simulink library "fm_lib"  (R2014a)
settings: Solver=ode45  SolverMode=SingleTasking  StartTime=0.0  StopTime=10.0  RelTol=1e-3
(part 2 of 2)

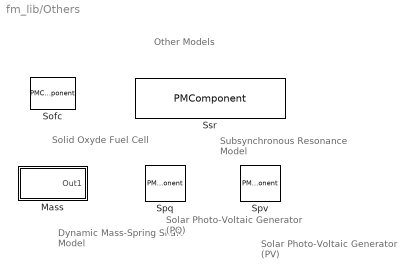
== system fm_lib/Others ==
  note: Other Models
  note: Subsynchronous
      | Resonance Model
  note: Solid Oxyde
      | Fuel Cell
  note: Dynamic Mass-Spring
      | Shaft Model
  note: Solar Photo-Voltaic
      | Generator (PQ)
  note: Solar Photo-Voltaic
      | Generator (PV)
  Mass : Subsystem  Tag=PSATblock  Description=Sparse Dynamic Component  mask(Mass){p2_3_4_5q=[0.6695  1.4612  1.6307  0.0903], p6_7_8_9q=[0.518  0.224  0.224  0.145], p10_11_12_13q=[0.0518  0.0224  0.0224  0.0145], p14_15_16_17q=[33.07  28.59  44.68  21.98], in=0, p18q=on}
      mask prompts: p2_3_4_5q "HP, IP, LP and EX inertiae [1/s 1/s 1/s 1/s]"; p6_7_8_9q "HP, IP, LP and EX damping [p.u. p.u. p.u. p.u.]"; p10_11_12_13q "D12, D23, D34 and D45 damping [p.u. p.u. p.u. p.u.]"; p14_15_16_17q "K12, K23, K34 and K45 coefficients"; in "Number of input signals"; p18q "Connected"
      mask help: This block defines a mechanical model for synchronous generator shaft.
      mask init:
      | fm_inout
      | [x,y] = fm_draw('circle');
      | [x1,y1] = fm_draw('semicircle');
      mask TypeOptions in: 0 | 1
      mask Callback p18q: fm_block
      mask Display: plot(-x1,y1,3+x,y,[0 3],[1 1],[0 3],[-1 -1],[3 5],[0 0])
  Sofc : PMComponent  Tag=PSATblock  Description=Sparse Dynamic Component  PhysicalDomain=psatdomain  LeftPortType=p1  RightPortType=p1  RConnTagsString=__newr0  mask(Sofc){p2_3q=[100  333.8], p4_13q=[0.8  5], p5_8_10q=[26.1  78.3  2.91], p6_9_11q=[8.43e-4  2.81e-4  2.52e-3], p7_17_12q=[0.996e-6  0.126  1.145], p14_15_16q=[0.85  0.9  0.8], p18_19q=[384  1.18], p20q=1273, p26q=0.1, p27_28q=[100  10], p29_30q=[1.2  0.8], p25q=0, p31q=on}
      mask prompts: p2_3q "DC Power and Voltage Rating [MW, kV]"; p4_13q "Electrical and fuel processor response times (Te, Tf) [s, s]"; p5_8_10q "Response times TH2, TH2O and TO2 [s, s, s]"; p6_9_11q "Valve molar constants KH2, KH2O and KO2"; p7_17_12q "Constant Kr, ohmic loss [Ohm] and hydrogen to oxygen ratio rH_O"; p14_15_16q "Fuel optimization constants Uopt, Umax and Umin"; p18_19q "Number of cells N0 and ideal standard potential E0 [V]"; p20q "Gas absolute temperature T [K]"; p26q "Transformer reactance Xt [p.u.]"; p27_28q "Gain and Time constant for Voltage Control Km, Tm [p.u.  s]"; p29_30q "Max and Min tap ratio [p.u./p.u. p.u./p.u.]"; p25q "Control Mode: [0] costant current; [1] costant power"; p31q "Connected"
      mask help: This block defines a Solid Oxyde Fuel Cell:
      mask TypeOptions p25q: 1 | 0
      mask Callback p31q: fm_block
      mask Display:
      | plot([0 1 1 0 0],[0 0 1 1 0])
      | plot([0.1 0.1 0.3 0.3],[1 1.1 1.1 1])
      | plot([0.9 0.9 0.7 0.7],[1 1.1 1.1 1])
      | color('yellow')
      | plot([0.85 0.75],[0.85 0.85],[0.15 0.25],[0.85 0.85],[0.8 0.8],[0.8 0.9])
      | color('blue')
      | plot([0.85 0.65 0.65 0.85 0.85],[0.3 0.3 0.7 0.7 0.3])
      | plot([0.15 0.15],[0.3 0.7],[0.35 0.35],[0.3 0.7],[0.15 0.35],[0.5 0.5])
      | plot([0.55 0.45 0.45 0.55 0.55 0.45],[0.15 0.15 0.25 0.25 0.35 0.35])
  Spq : PMComponent  Tag=PSATblock  Description=Sparse Dynamic Component  PhysicalDomain=psatdomain  LeftPortType=p1  RightPortType=p1  RConnTagsString=__newr0  mask(Spq){p2_3q=[60  80], p4_5q=[15  15], p6q=on}
      mask prompts: p2_3q "Active and Reactive Power Rating [MW, MVar]"; p4_5q "Inverter response times (Tp, Tq) [s, s]"; p6q "Connected"
      mask help: This block defines a Solar Photo-Voltaic generator with constant PQ model.
      mask init:
      | [x,y] = fm_draw('circle');
      | [xc,yc] = fm_draw('S');
      mask Callback p6q: fm_block
      mask Display:
      | plot(x,y,[-0.25 -0.25],[-0.25 0.25])
      | color('blue')
      | plot(xc,yc)
  Spv : PMComponent  Tag=PSATblock  Description=Sparse Dynamic Component  PhysicalDomain=psatdomain  LeftPortType=p1  RightPortType=p1  RConnTagsString=__newr0  mask(Spv){p2_3q=[40  1.045], p4_5q=[0.015  0.015], p6_7q=[0.0868  50.9005], p8q=on}
      mask prompts: p2_3q "Active Power and Voltage References [MW, p.u.]"; p4_5q "Inverter response times (Tp, Tq) [s, s]"; p6_7q "Voltage PI Controller Gains (kv, ki)"; p8q "Connected"
      mask help:
      | This block defines a Solar Photo-Voltaic generator.
      | P_ref = const
      | V_ref = const
      mask init:
      | [x,y] = fm_draw('circle');
      | [x1,y1] = fm_draw('sunedge');
      | [xp,yp] = fm_draw('G');
      mask Callback p8q: fm_block
      mask Display:
      | plot(1.1*x,1.1*y,[-0.25 -0.25],[-0.25 0.25])
      | plot(1.5*x1,y1)
      | plot(-1.5*x1,y1)
      | plot(y1,1.5*x1)
      | plot(y1,-1.5*x1)
      | color('blue')
      | plot(0.5*xp,0.5*yp)
  Ssr : PMComponent  Tag=PSATblock  Description=Sparse Dynamic Component  PhysicalDomain=psatdomain  LeftPortType=p1  RightPortType=p1  RConnTagsString=__newr0  mask(SSR){p2_3_4q=[100   230  60], p5_6q=[1.79  1.71], p8_7q=[1.66  0.015], p13_12q=[1.70  0.01], p9_10_11q=[0.0165  0.30  0.05], p14_15_16_17_18q=[0.6695  1.4612  1.6307  1.5228  0.0903], p19_20_21_22_23q=[0.518  0.224  0.224  0.000  0.145], p24_25_26_27q=[33.07  28.59  44.68  21.98], p28q=on}
      mask prompts: p2_3_4q "Power, Voltage and Frequency Ratings [MVA, kV, Hz]"; p5_6q "Machine reactances Xd, Xq [p.u. p.u.]"; p8_7q "Armature parameters Xad, Ra [p.u. p.u.]"; p13_12q "D-axis parameters Xf, Rf [p.u. p.u.]"; p9_10_11q "Line parameters R, Xl, Xc [p.u. p.u. p.u.]"; p14_15_16_17_18q "Inertiae M (HP, IP, LP, rotor, EX)"; p19_20_21_22_23q "Dampings D (HP, IP, LP, rotor, EX)"; p24_25_26_27q "Shaft coefficients K12, K23, K34, K45"; p28q "Connected"
      mask help: This block defines a fourth order synchronous machine with shaft dynamics and compensated line.
      mask init:
      | [x,y] = fm_draw('circle');
      | [xg,yg] = fm_draw('G');
      | [xs,ys] = fm_draw('sinus');
      mask Callback p28q: fm_block
      mask Display:
      | plot(0,-50,450,50,[0 30 30 38 53 68 83 98 113 120 120 150],[0 0 0 25 -25 25 -25 25 -25 0 0 0],[0 23 23 24 28 34 40 47 52 55 56 54 51 51 47 46 48 51 57 64 70 75 79 79 77 74 74 70 69 71 75 80 87 93 99 102 103 101 97 97 94 93 94 98 104 110 117 122 125 126 126 150]+150,[0 0 1 11 19 24 25 23 17 8 -2 -12 -18 -18 -9 1 11 19 24 25 23 17 8 -2 -12 -18 -18 -9 1 11 19 24 25 23 17 8 -2 -12 -18 -18 -9 1 11 19 24 25 23 17 8 0 0 0],[0 60 60 57 55 57 60 60 57 55]+300,[0 0 8 16 25 16 8 -8 -16 -25],[90 90 90 150]+300,[25 -25 0 0])
      | plot(-150+60*(x+1.4),40*y,-150+60*0.12*xs+60,40*0.15*ys-40*0.6)
      | color('blue')
      | plot(-150+60*0.45*(xg+1.4)+60*0.75,40*0.45*yg+40*0.3)

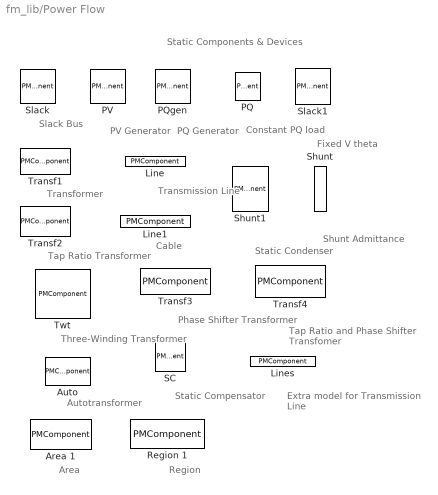
== system fm_lib/Power Flow ==
  note: Static Components & Devices
  note: Slack Bus
  note: PV
      | Generator
  note: Constant
      | PQ load
  note: Transmission
      | Line
  note: Transformer
  note: Shunt
      | Admittance
  note: Tap Ratio
      | Transformer
  note: Phase Shifter
      | Transformer
  note: Tap Ratio and
      | Phase Shifter
      | Transfomer
  note: Extra model for
      | Transmission Line
  note: Static
      | Compensator
  note: Autotransformer
  note: Static
      | Condenser
  note: Cable
  note: Three-Winding
      | Transformer
  note: PQ
      | Generator
  note: Fixed V
      | theta
  note: Area
  note: Region
  Area 1 : PMComponent  Tag=PSATblock  Description=Power Flow  PhysicalDomain=psatdomain  LeftPortType=p1  RightPortType=p1  mask(Areas){out=0, p1q=1, p2q=0, p3q=100, p4q=0, p5q=0.01, p6q=0, p7_8q=[0  0]}
      mask prompts: out "Output for slack bus connection"; p1q "Area Id Number (must be unique)"; p2q "Slack bus number (can be zero)"; p3q "Power rating [MVA]"; p4q "Power interchange export (>0 = out) [p.u.]"; p5q "Power interchange tolerance [p.u.]"; p6q "Annual growth rate [%]"; p7_8q "Actual net interchange powers P and Q [p.u.]"
      mask help: Area block.
      mask init:
      | fm_inout
      | [xc,yc] = fm_draw('rounded');
      settings: CopyFcn=idnum(Areas,gcb,gcs)
      mask TypeOptions out: 0 | 1
      mask Callback out: fm_block
      mask Callback p1q: fm_block
      mask Display: plot(xc,yc), color('blue'), text(-0.5,0.1,'Area 1')
  Auto : PMComponent  Tag=PSATblock  Description=Power Flow  PhysicalDomain=psatdomain  LeftPortType=p1  RightPortType=p1  LConnTagsString=__newl0  RConnTagsString=__newr0  mask(Line){p3_4_5q=[100  400 60], p7q=1, p8q=0.01, p9q=0.20, p13_14_15q=[0.0  0.0  0.0], p16q=on}
      mask prompts: p3_4_5q "Power, Voltage and Frequency Ratings [MVA, kV, Hz]"; p7q "Primary and secondary voltage ratio [kV/kV]"; p8q "Resistance [p.u.]"; p9q "Reactance [p.u.]"; p13_14_15q "Imax, Pmax and Smax [p.u., p.u., p.u.]"; p16q "Connected"
      mask help: This block defines an auto-transformer.
      mask init:
      | [x,y] = fm_draw('circle');
      | [xq,yq] = fm_draw('quarter');
      mask Callback p16q: fm_block
      mask Display: plot(x,y,1.75*xq,yq,[-1 -1.3],[0 0],[1.75 2.05],[0 0])
  Line : PMComponent  Tag=PSATblock  Description=Power Flow  PhysicalDomain=psatdomain  LeftPortType=p1  RightPortType=p1  LConnTagsString=__newl0  RConnTagsString=__newr0  mask(Line){p3_4_5q=[100  400  60], p6q=0, p8q=0.01, p9q=0.10, p10q=1e-3, p13_14_15q=[0.0  0.0  0.0], p16q=on}
      mask prompts: p3_4_5q "Power, Voltage and Frequency Ratings [MVA, kV, Hz]"; p6q "Length of line [km] (0 for p.u. parameters)"; p8q "Resistance [p.u. (Ohms/km)]"; p9q "Reactance [p.u. (H/km)]"; p10q "Susceptance [p.u. (F/km)]"; p13_14_15q "Imax, Pmax and Smax [p.u., p.u., p.u.]"; p16q "Connected"
      mask help: This block defines a pi model for a tree phase line.
      mask init:
      | [xp,yp] = fm_draw('pi');
      mask Callback p16q: fm_block
      mask Display:
      | plot([-1  1  1 -1 -1],[-0.2 -0.2 0.2 0.2 -0.2])
      | color('blue')
      | plot(0.35*xp,0.2*yp)
  Line1 : PMComponent  Tag=PSATblock  Description=Power Flow  PhysicalDomain=psatdomain  LeftPortType=p1  RightPortType=p1  LConnTagsString=__newl0  RConnTagsString=__newr0  mask(Line){p3_4_5q=[100  400  60], p6q=0, p8q=0.01, p9q=0.10, p10q=1e-3, p13_14_15q=[0.0  0.0  0.0], p16q=on}
      mask prompts: p3_4_5q "Power, Voltage and Frequency Ratings [MVA, kV, Hz]"; p6q "Length of line [km] (0 for p.u. parameters)"; p8q "Resistance [p.u. (Ohms/km)]"; p9q "Reactance [p.u. (H/km)]"; p10q "Susceptance [p.u. (F/km)]"; p13_14_15q "Imax, Pmax and Smax [p.u., p.u., p.u.]"; p16q "Connected"
      mask help: This block defines a pi model for a tree phase cable.
      mask init:
      | [x,y] = fm_draw('circle');
      | [x1,y1] = fm_draw('semicircle');
      mask Callback p16q: fm_block
      mask Display:
      | color('yellow')
      | plot(10+0.433*x,0.5+0.433*y)
      | plot(9.567+0.433*x,-0.25+0.433*y)
      | plot(10.433+0.433*x,-0.25+0.433*y)
      | color('black')
      | plot(-x1,y1)
      | plot(10+x,y,[0 10],[1 1],[0 10],[-1 -1])
  Lines : PMComponent  Tag=PSATblock  Description=Power Flow  PhysicalDomain=psatdomain  LeftPortType=p1  RightPortType=p1  LConnTagsString=__newl0  RConnTagsString=__newr0  mask(Lines){p3_4_5q=[100  400  60], p6_7_8q=[0.01  0.10  0.00], p9q=on}
      mask prompts: p3_4_5q "Power, Voltage and Frequency Ratings [MVA, kV, Hz]"; p6_7_8q "Resistance, Reactance and Susceptance [p.u.  p.u.  p.u.]"; p9q "Connected"
      mask help:
      | This block defines a pi model for a tree phase line.
      | The line is NOT included in the admittance matrix.
      mask init:
      | [xp,yp] = fm_draw('L');
      mask Callback p9q: fm_block
      mask Display:
      | plot([-1  1  1 -1 -1],[-0.2 -0.2 0.2 0.2 -0.2])
      | color('blue')
      | plot(0.35*xp,0.2*yp)
  PQ : PMComponent  Tag=PSATblock  Description=Power Flow  PhysicalDomain=psatdomain  LeftPortType=p1  RightPortType=p1  LConnTagsString=__newl0  mask(PQ){p2_3q=[100  400], p4_5q=[0.80  0.60], p6_7q=[1.2  0.8], p8q=on, p9q=on}
      mask prompts: p2_3q "Power and Voltage Ratings [MVA, kV]"; p4_5q "Active and Reactive Powers [p.u.  p.u.]"; p6_7q "Maximum and Minimum Allowable Voltage [p.u.   p.u.]"; p8q "Allow conversion to impendance for min or max voltage"; p9q "Connected"
      mask help:
      | This block defines a constant power load:
      |
      | P = Pcost.
      | Q = Qcost.
      mask Callback p8q: fm_block
      mask Callback p9q: fm_block
      mask Display: plot([1 -0.5 -0.5 1],[0 0.866 -0.866 0])
  PQgen : PMComponent  Tag=PSATblock  Description=Power Flow  PhysicalDomain=psatdomain  LeftPortType=p1  RightPortType=p1  RConnTagsString=__newr0  mask(PQgen){p2_3q=[100  400], p4_5q=[0.8  0.6], p6_7q=[1.1  0.9], p8q=off, p9q=on}
      mask prompts: p2_3q "Power and Voltage Ratings [MVA, kV]"; p4_5q "Active and Reactive Powers [p.u.  p.u.]"; p6_7q "Vmax and Vmin [p.u.  p.u.]"; p8q "Allow conversion to impedance"; p9q "Connected"
      mask help: This block defines a PQ generator.
      mask init:
      | [x,y] = fm_draw('circle');
      | [xp,yp] = fm_draw('P');
      | [xq,yq] = fm_draw('Q');
      mask Callback p8q: fm_block
      mask Callback p9q: fm_block
      mask Display:
      | plot(x,y)
      | color('blue')
      | plot(0.3*xp-0.35,0.6*yp,0.4*xq+0.1,0.6*yq)
  PV : PMComponent  Tag=PSATblock  Description=Power Flow  PhysicalDomain=psatdomain  LeftPortType=p1  RightPortType=p1  RConnTagsString=__newr0  mask(PV){p2_3q=[100  400], p4q=0.8, p5q=1.00, p6_7q=[0.8  -0.2], p8_9q=[1.1  0.9], p10q=1, p11q=on}
      mask prompts: p2_3q "Power and Voltage Ratings [MVA, kV]"; p4q "Active Power [p.u.]"; p5q "Voltage Magnitude [p.u.]"; p6_7q "Qmax and Qmin [p.u.  p.u.]"; p8_9q "Vmax and Vmin [p.u.  p.u.]"; p10q "Loss Participation Factor"; p11q "Connected"
      mask help:
      | This block defines a PV bus for load flow studies:
      |
      | P = Pcost.
      | V = Vdes.
      mask init:
      | [x,y] = fm_draw('circle');
      | [xp,yp] = fm_draw('P');
      mask Callback p11q: fm_block
      mask Display:
      | plot(x,y)
      | color('blue')
      | plot(0.3*xp-0.35,0.6*yp,[0.1 0.3 0.5],[0.3 -0.3 0.3])
  Region 1 : PMComponent  Tag=PSATblock  Description=Power Flow  PhysicalDomain=psatdomain  LeftPortType=p1  RightPortType=p1  mask(Regions){out=0, p1q=1, p2q=0, p3q=100, p4q=0, p5q=0.01, p6q=0, p7_8q=[0  0]}
      mask prompts: out "Output for slack bus connection"; p1q "Region Id Number (must be unique)"; p2q "Slack bus number (can be zero)"; p3q "Power rating [MVA]"; p4q "Power interchange export (>0 = out) [p.u.]"; p5q "Power interchange tolerance [p.u.]"; p6q "Annual growth rate [%]"; p7_8q "Actual net interchange powers P and Q [p.u.]"
      mask help: Region block.
      mask init:
      | fm_inout
      | [xc,yc] = fm_draw('rounded');
      settings: CopyFcn=idnum(Regions,gcb,gcs)
      mask TypeOptions out: 0 | 1
      mask Callback out: fm_block
      mask Callback p1q: fm_block
      mask Display: plot(xc,yc), color('blue'), text(-0.5,0.1,'Region 1')
  SC : PMComponent  Tag=PSATblock  Description=Power Flow  PhysicalDomain=psatdomain  LeftPortType=p1  RightPortType=p1  RConnTagsString=__newr0  mask(PV){p2_3q=[100  400], p5q=1.00, p6_7q=[0.8  -0.2], p8_9q=[1.1  0.9], p10q=1, p11q=on}
      mask prompts: p2_3q "Power and Voltage Ratings [MVA, kV]"; p5q "Voltage Magnitude [p.u.]"; p6_7q "Qmax and Qmin [p.u.  p.u.]"; p8_9q "Vmax and Vmin [p.u.  p.u.]"; p10q "Loss Participation Coefficient"; p11q "Connected"
      mask help:
      | This block defines a static synchronous compensator:
      | P = 0
      | V = Vdes
      mask init:
      | [x,y] = fm_draw('circle');
      | [xc,yc] = fm_draw('C');
      mask Callback p11q: fm_block
      mask Display:
      | plot(x,y,[-0.25 -0.25],[-0.25 0.25])
      | color('blue')
      | plot(0.5*xc-0.25,yc)
  Shunt : PMComponent  Tag=PSATblock  Description=Power Flow  PhysicalDomain=psatdomain  LeftPortType=p1  RightPortType=p1  LConnTagsString=__newl0  mask(Shunt){p2_3_4q=[100  400 60], p5_6q=[0.0  0.5], p7q=on}
      mask prompts: p2_3_4q "Power, Voltage and Frequency Ratings [MVA, kV, Hz]"; p5_6q "Conductance G and Susceptance B [p.u.  p.u.]"; p7q "Connected"
      mask help: This block defines a constant admittance.
      mask init:
      | [xp,yp] = fm_draw('Y');
      mask Callback p5_6q: fm_block
      mask Callback p7q: fm_block
      mask Display:
      | plot([-1 1 1 -1 -1],[0.2 0.2 -0.2 -0.2 0.2])
      | plot([-1  -1.5],[0 0],[1 1.2],[0 0],[1.2 1.2],[-0.2 0.2],[1.35 1.35],[-0.125 0.125],[1.5 1.5],[-0.05 0.05])
      | color('blue')
      | plot(xp,0.3*yp)
  Shunt1 : PMComponent  Tag=PSATblock  Description=Power Flow  PhysicalDomain=psatdomain  LeftPortType=p1  RightPortType=p1  LConnTagsString=__newl0  mask(Shunt){p2_3_4q=[100  400  60], p6q=0.5, p7q=on}
      mask prompts: p2_3_4q "Power, Voltage and Frequency Ratings [MVA, kV, Hz]"; p6q "Susceptance B [p.u.]"; p7q "Connected"
      mask help:
      | This block defines a static condenser:
      |
      | Q = B * V^2
      |
      | (Negative values of B define an inductive load).
      mask init:
      | fm_block
      mask Callback p7q: fm_block
      mask Display: plot(-[0 60 60 55 53 55 60 60 55 53]/150,[0 0 8 16 25 16 8 -8 -16 -25]/50,-[80 80 80 150]/150,[25 -25 0 0]/50,[0 0],[-0.4 0.4],[0.075 0.075],[-0.25 0.25],[0.15 0.15],[-0.1 0.1])
  Slack : PMComponent  Tag=PSATblock  Description=Power Flow  PhysicalDomain=psatdomain  LeftPortType=p1  RightPortType=p1  RConnTagsString=__newr0  mask(SW){p2_3q=[100  400], p4q=1.00, p5q=0.00, p6_7q=[1.5  -1.5], p8_9q=[1.1  0.9], p10q=0.80, p11q=1, p12q=on, p13q=on}
      mask prompts: p2_3q "Power and Voltage Ratings [MVA, kV]"; p4q "Voltage Magnitude [p.u.]"; p5q "Reference Phase Angle [rad]"; p6_7q "Qmax and Qmin [p.u.  p.u.]"; p8_9q "Vmax and Vmin  [p.u.  p.u.]"; p10q "Active Power Guess [p.u.]"; p11q "Loss Participation Factor"; p12q "Reference bus"; p13q "Connected"
      mask help:
      | This block defines a V-theta bus:
      |
      | V = V_des
      | theta = theta_des
      mask init:
      | [x,y] = fm_draw('circle');
      | [xt,yt] = fm_draw('theta');
      mask Callback p12q: fm_block
      mask Callback p13q: fm_block
      mask Display: plot([0 1 1 0 0],[0 0 1 1 0]), color('blue'), plot([0 1],[0 1],[0 1],[1 0],[0.5 1 0.5 0 0.5],[0 0.5 1 0.5 0])
  Slack1 : PMComponent  Tag=PSATblock  Description=Power Flow  PhysicalDomain=psatdomain  LeftPortType=blob  RightPortType=blob  RConnTagsString=__newr0  mask(SW){p2_3q=[100  400], p4q=1.00, p5q=0.00, p6_7q=[1.5  -1.5], p8_9q=[1.1  0.9], p10q=0.80, p11q=1, p12q=off, p13q=on}
      mask prompts: p2_3q "Power and Voltage Ratings [MVA, kV]"; p4q "Voltage Magnitude [p.u.]"; p5q "Reference Phase Angle [rad]"; p6_7q "Qmax and Qmin [p.u.  p.u.]"; p8_9q "Vmax and Vmin  [p.u.  p.u.]"; p10q "Active Power Guess [p.u.]"; p11q "Loss Participation Factor"; p12q "Reference bus"; p13q "Connected"
      mask help:
      | This block defines a V-theta bus:
      |
      | V = V_des
      | theta = theta_des
      mask init:
      | [x,y] = fm_draw('circle');
      | [xt,yt] = fm_draw('theta');
      mask Callback p12q: fm_block
      mask Callback p13q: fm_block
      mask Display:
      | plot(x,y)
      | color('blue')
      | plot([0.1 0.3 0.5]-0.6,[0.3 -0.3 0.3],0.45*xt+0.1,0.6*yt)
  Transf1 : PMComponent  Tag=PSATblock  Description=Power Flow  PhysicalDomain=psatdomain  LeftPortType=p1  RightPortType=p1  LConnTagsString=__newl0  RConnTagsString=__newr0  mask(Line){p3_4_5q=[100  400  60], p7q=1, p8q=0.01, p9q=0.20, p13_14_15q=[0.0  0.0  0.0], p16q=on}
      mask prompts: p3_4_5q "Power, Voltage and Frequency Ratings [MVA, kV, Hz]"; p7q "Primary and secondary voltage ratio [kV/kV]"; p8q "Resistance [p.u.]"; p9q "Reactance [p.u.]"; p13_14_15q "Imax, Pmax and Smax [p.u., p.u., p.u.]"; p16q "Connected"
      mask help: This block defines a transformer.
      mask init:
      | [x,y] = fm_draw('circle');
      | [x1,y1] = fm_draw('1');
      | [x2,y2] = fm_draw('2');
      mask Callback p16q: fm_block
      mask Display:
      | plot(x,y,x+1.4,y,[-1 -1.3],[0 0],[2.4 2.7],[0 0])
      | color('green')
      | plot(-0.1+0.65*x1,0.65*y1)
      | plot(1.5+0.65*x2,0.65*y2)
  Transf2 : PMComponent  Tag=PSATblock  Description=Power Flow  PhysicalDomain=psatdomain  LeftPortType=p1  RightPortType=p1  LConnTagsString=__newl0  RConnTagsString=__newr0  mask(Line){p3_4_5q=[100  400  60], p7q=400/400, p8q=0.01, p9q=0.20, p11q=1.00, p13_14_15q=[0.0  0.0  0.0], p16q=on}
      mask prompts: p3_4_5q "Power, Voltage and Frequency Ratings [MVA, kV, Hz]"; p7q "Primary and secondary voltage ratio [kV/kV]"; p8q "Resistance [p.u.]"; p9q "Reactance [p.u.]"; p11q "Fixed tap ratio [p.u./p.u.]"; p13_14_15q "Imax, Pmax and Smax  [p.u., p.u., p.u.]"; p16q "Connected"
      mask help: This block defines a transformer with constant tap ratio.
      mask init:
      | [x,y] = fm_draw('circle');
      | [x2,y2] = fm_draw('2');
      mask Callback p16q: fm_block
      mask Display:
      | plot(x,y,x+1.4,y,[-1 -1.3],[0 0],[2.4 2.7],[0 0])
      | color('green')
      | plot([-0.8 0.7],[-1.2 1.2],[0.5 0.7],[1.1 1.2],[0.7 0.7],[1.0 1.2])
      | plot(1.5+0.65*x2,0.65*y2)
  Transf3 : PMComponent  Tag=PSATblock  Description=Power Flow  PhysicalDomain=psatdomain  LeftPortType=p1  RightPortType=p1  LConnTagsString=__newl0  RConnTagsString=__newr0  mask(Line){p3_4_5q=[100  400 60], p7q=400/400, p8q=0.01, p9q=0.20, p12q=0.00, p13_14_15q=[0.0  0.0  0.0], p16q=on}
      mask prompts: p3_4_5q "Power, Voltage and Frequency Ratings [MVA, kV, Hz]"; p7q "Primary and secondary voltage ratio [kV/kV]"; p8q "Resistance [p.u.]"; p9q "Reactance [p.u.]"; p12q "Fixed phase shift [deg]"; p13_14_15q "Imax, Pmax and Smax [p.u. p.u. p.u.]"; p16q "Connected"
      mask help: This block defines a transformer with constant phase shifter.
      mask init:
      | [x,y] = fm_draw('circle');
      | [xa,ya] = fm_draw('a');
      | [x1,y1] = fm_draw('1');
      | [x2,y2] = fm_draw('2');
      mask Callback p16q: fm_block
      mask Display:
      | plot(x,y,x+1.4,y,[-1 -1.3],[0 0],[2.4 2.7],[0 0],[2.7 2.7 4 4 2.7],[-0.5 0.5 0.5 -0.5 -0.5],[4 4.3],[0 0])
      | color('red')
      | plot(3.35+0.2*xa,-0.1+0.15*ya)
      | color('green')
      | plot(-0.1+0.65*x1,0.65*y1)
      | plot(1.5+0.65*x2,0.65*y2)
  Transf4 : PMComponent  Tag=PSATblock  Description=Power Flow  PhysicalDomain=psatdomain  LeftPortType=p1  RightPortType=p1  LConnTagsString=__newl0  RConnTagsString=__newr0  mask(Line){p3_4_5q=[100  400  60], p7q=400/400, p8q=0.01, p9q=0.20, p11q=1.00, p12q=0.00, p13_14_15q=[0.0  0.0  0.0], p16q=on}
      mask prompts: p3_4_5q "Power, Voltage and Frequency Ratings [MVA, kV, Hz]"; p7q "Primary and secondary voltage ratio [kV/kV]"; p8q "Resistance [p.u.]"; p9q "Reactance [p.u.]"; p11q "Fixed tap ratio [p.u./p.u.]"; p12q "Fixed phase shift [deg]"; p13_14_15q "Imax, Pmax and Smax [p.u. p.u. p.u.]"; p16q "Connected"
      mask help: This block defines a transformer with constant phase shifter and constant tap ratio.
      mask init:
      | [x,y] = fm_draw('circle');
      | [xa,ya] = fm_draw('a');
      | [x2,y2] = fm_draw('2');
      mask Callback p16q: fm_block
      mask Display:
      | plot(x,y,x+1.4,y,[-1 -1.3],[0 0],[2.4 2.7],[0 0],[2.7 2.7 4 4 2.7],[-0.5 0.5 0.5 -0.5 -0.5],[4 4.3],[0 0])
      | color('green')
      | plot([-0.8 0.7],[-1.2 1.2],[0.5 0.7],[1.1 1.2],[0.7 0.7],[1.0 1.2])
      | plot(1.5+0.65*x2,0.65*y2)
      | color('red')
      | plot(3.35+0.2*xa,-0.1+0.15*ya)
  Twt : PMComponent  Tag=PSATblock  Description=Power Flow  PhysicalDomain=psatdomain  LeftPortType=p1  RightPortType=p1  LConnTagsString=__newl0  RConnTagsString=__newr0|__newr1  mask(Twt){p4_5q=[100  60], p6_7_8q=[230 132 60], p9_10_11q=[0.01 0.01 0.01], p12_13_14q=[0.1 0.1 0.1], p15q=1.00, p16_17_18q=[0.0  0.0  0.0], p19_20_21q=[0.0  0.0  0.0], p22_23_24q=[0.0  0.0  0.0], p25q=on}
      mask prompts: p4_5q "Power and Frequency Ratings [MVA, Hz]"; p6_7_8q "Voltage Ratings Vn1, Vn2 and Vn3 [kV, kV, kV]"; p9_10_11q "Resistances R12, R13 and R23 [p.u.  p.u.  p.u.]"; p12_13_14q "Reactances X12, X13 and X23 [p.u.  p.u.  p.u.]"; p15q "Fixed tap ratio [p.u./p.u.]"; p16_17_18q "Max Currents Imax1, Imax2 and Imax3  [p.u. p.u. p.u.]"; p19_20_21q "Max Powers Pmax1, Pmax2 and Pmax3 [p.u. p.u. p.u.]"; p22_23_24q "Max Powers Smax1, Smax2 and Smax3 [p.u. p.u. p.u.]"; p25q "Connected"
      mask help: This block defines a three-winding transformer with constant tap ratio.
      mask init:
      | [x,y] = fm_draw('circle');
      | [x2,y2] = fm_draw('2');
      | [x3,y3] = fm_draw('3');
      mask Callback p25q: fm_block
      mask Display:
      | plot(x,y,x+1.4,0.8+y,1.4+x,y-0.8,[-1 -1.3],[0 0],[2.4 2.75],[0.9 0.9],[2.4 2.75],[-0.9 -0.9])
      | color('green')
      | plot([-0.8 0.7]-0.4,[-1.2 1.2]+0.2,[0.5 0.7]-0.4,[1.1 1.2]+0.2,[0.7 0.7]-0.4,[1.0 1.2]+0.2)
      | plot(1.5+0.65*x2,0.9+0.65*y2)
      | plot(1.5+0.65*x3,-0.9+0.65*y3)

== system fm_lib/ULTC ==
  note: Regulating Transformers
  note: Under Load Tap
      | Changer with
      | Embedded Load
  note: Under Load Tap
      | Changer
  note: Phase Shifting
      | Transformer
  note: Under Load Tap
      | Changer with
      | Remote Voltage Control
  Ltc : Subsystem  Tag=PSATblock  Description=ULTC  mask(Ltc){p3_5q=[100  60], p4_6q=[220   5], p16q=1, p8_7q=[0.10  1e-3], p9_10q=[1.20  0.8], p11q=0, p12q=1.00, p14_13q=[0.10  0.001], p17q=5, p18q=on}
      mask prompts: p3_5q "Power and Frequency ratings [MVA, Hz]"; p4_6q "Primary Voltage rating and nominal tap ratio V1/V2 [kV,  kV/kV]"; p16q "Control Type"; p8_7q "Inverse Time Constant and integral deviation [1/s, p.u.]"; p9_10q "Max and Min Tap Ratio [p.u./p.u.  p.u./p.u.]"; p11q "Tap ratio step [0 for continuous model]"; p12q "Reference Voltage Vref [p.u.]"; p14_13q "Resistance and Reactance  [p.u.  p.u.]"; p17q "Dead zone [%]"; p18q "Connected"
      mask help:
      | This block defines a pi model for a LTC Transformer.
      |
      | Control type:
      |
      | [1] secondary V control;
      | [2] secondary Q control;
      | [3] remote V control.
      mask init:
      | rot = strcmp(get_param(gcb,'NamePlacement'),'normal');
      | [x,y] = fm_draw('circle');
      mask TypeOptions p16q: 1 | 2 | 3
      mask Callback p16q: fm_block
      mask Callback p18q: fm_block
      mask Display: plot(x,y,x+1.4,y,[2.4 2.8],[0 0],[3.1 3.5],[0 0],[-1 -2],[0 0],0,2), color('green'), plot([2.95 2.95],[-0.15 -2],[2.95 -0.8],[-2 -2],[-0.8 -0.8],[-2 -1.2], [-0.8 0.7],[-1.2 1.2],[0.5 0.7],[1.1 1.2],[0.7 0.7], [1.0 1.2],[2.8 3.1 3.1 2.8 2.8],[-0.15 -0.15 0.15 0.15 -0.15]);
  Ltc1 : Subsystem  Tag=PSATblock  Description=ULTC  mask(Ltc){p3_5q=[100  60], p4_6q=[220   5], p16q=3, p8_7q=[0.10  1e-3], p9_10q=[1.20  0.8], p11q=0, p12q=1.00, p14_13q=[0.10  0.001], p17q=5, p18q=on}
      mask prompts: p3_5q "Power and Frequency ratings [MVA, Hz]"; p4_6q "Primary Voltage rating and nominal tap ratio V1/V2 [kV,  kV/kV]"; p16q "Control Type"; p8_7q "Inverse Time Constant and integral deviation [1/s, p.u.]"; p9_10q "Max and Min Tap Ratio [p.u./p.u.  p.u./p.u.]"; p11q "Tap ratio step [0 for continuous model]"; p12q "Remote Reference Voltage Vref [p.u.]"; p14_13q "Resistance and Reactance  [p.u.  p.u.]"; p17q "Dead zone [%]"; p18q "Connected"
      mask help:
      | This block defines a pi model for a LTC Transformer.
      |
      | Control type:
      |
      | [1] secondary V control;
      | [2] secondary Q control;
      | [3] remote V control.
      mask init:
      | rot = strcmp(get_param(gcb,'NamePlacement'),'normal');
      | [x,y] = fm_draw('circle');
      mask TypeOptions p16q: 1 | 2 | 3
      mask Callback p16q: fm_block
      mask Callback p18q: fm_block
      mask Display: plot(x,y,x+1.4,y,[2.4 3.5],[0 0],[-1 -2],[0 0],0,2-4*rot), color('green'), plot([0.8 0.8],3*rot-[1.3 1.7],[0.65 0.95 0.95 0.65 0.65],[3.4*rot-1.7 3.4*rot-1.7 4*rot-2 4*rot-2 3.4*rot-1.7],[0.8 -0.8],[2.4*rot-1.2 1.3-2.6*rot],[-0.6 -0.8],[1.1-2.2*rot 1.2-2.4*rot],[-0.8 -0.8], [1-2*rot 1.2-2.4*rot]);
  Phs : PMComponent  Tag=PSATblock  Description=Phase Shifter  PhysicalDomain=psatdomain  LeftPortType=p1  RightPortType=p1  LConnTagsString=__newl0  RConnTagsString=__newr0  mask(Phs){p3_6q=[100  60], p4_5q=[230  138], p7q=0.001, p13_14q=[pi/2  -pi/2], p8_9q=[0.05  0.1], p10q=1.00, p11_12q=[0.01  0.1], p15q=1, p16q=on}
      mask prompts: p3_6q "Power and Frequency ratings [MVA, Hz]"; p4_5q "Primary and Secondary Voltage ratings [kV,  kV]"; p7q "Time constant of measurement block [s]"; p13_14q "Max and Min Phase angle [rad rad]"; p8_9q "Proportional and Integral Gains [Kp Ki]"; p10q "Reference Power Pref [p.u.]"; p11_12q "Resistance and Reactance  [p.u.  p.u.]"; p15q "Tap ratio [p.u./p.u.]"; p16q "Connected"
      mask help: This block defines a pi model for a Phase Shifting Transformer.
      mask init:
      | if strcmp(get_param(gcb,'NamePlacement'),'alternate'), rot = 0; else, rot = 1; end
      | [x,y] = fm_draw('circle');
      | [xa,ya] = fm_draw('a');
      mask Callback p16q: fm_block
      mask Display:
      | plot(x,y,x+1.4,y,[-1 -1.3],[0 0],[2.4 2.7],[0 0],[2.7 2.7 4 4 2.7],[-0.5 0.5 0.5 -0.5 -0.5],[4 4.3],[0 0],[-1.7 -2],[0 0])
      | color('green')
      | plot([-1.3 -1.3 -1.7 -1.7 -1.3],[0.2 -0.2 -0.2 0.2 0.2],[3.35 3.35 -1.5 -1.5],[-0.5 -2 -2 -0.2],0,2)
      | color('red')
      | plot(3.35+0.2*xa,-0.1+0.15*ya)
  Tap : PMComponent  Tag=PSATblock  Description=ULTC  PhysicalDomain=psatdomain  LeftPortType=p1  RightPortType=p1  LConnTagsString=__newl0  mask(Tap){p2_3q=[100  60], p4q=1e-3, p5q=0.10, p6_7q=[1.20  0.80], p8q=1.00, p9_10q=[0.80  0.60], p11_12q=[2.00  2.00], p13q=on}
      mask prompts: p2_3q "Power and Voltage Ratings [MVA, kV]"; p4q "Integral Behaviour Deviation"; p5q "Inverse Time Constant [1/s]"; p6_7q "Max and Min Tap Ratio Limits [p.u./p.u.  p.u./p.u.]"; p8q "Reference Voltage [p.u.]"; p9_10q "Nominal Active and Reactive Power Ratings [p.u.  p.u.]"; p11_12q "Active and Reactive Power Exponents"; p13q "Connected"
      mask help: This block defines an ideal LTC transformer feeding a static load described by monomial expressions.
      mask init:
      | [x,y] = fm_draw('circle');
      mask Callback p13q: fm_block
      mask Display:
      | plot(x,y,x+1.4,y)
      | plot([-1 -1.3],[0 0],[2.4 2.8],[0 0],[3.1 3.7],[0 0],0,2)
      | plot([3.7 3.7 5.7 5.7 3.7],[-1 1 1 -1 -1])
      | color('green')
      | plot([-0.8 0.7],[-1.2 1.2],[0.5 0.7],[1.1 1.2],[0.7 0.7],[1.0 1.2])
      | plot([2.8 3.1 3.1 2.8 2.8],[-0.15 -0.15 0.15 0.15 -0.15])
      | plot([2.95 2.95],[-0.15 -2],[2.95 -0.8],[-2 -2],[-0.8 -0.8],[-2 -1.2])
      | color('blue')
      | plot([4.2 4.2 5.2],[0.6 -0.6 -0.6])

== system fm_lib/Wind Turbines ==
  note: Constant Speed
      | Wind Turbine with
      | Squirrel Cage
      | Induction Generator
  note: Wind Turbines
  note: Wind Model
  note: Variable Speed
      | Wind Turbine with
      | Doubly Fed Induction
      | Generator
  note: Variable Speed
      | Wind Turbine with
      | Direct Drive Synchronous
      | Generator
  Cswt : PMComponent  Tag=PSATblock  Description=Wind Turbines  PhysicalDomain=psatdomain  LeftPortType=p1  RightPortType=p1  LConnTagsString=__newl0  RConnTagsString=__newr0  mask(Cswt){p3_4_5q=[2   25   60], p6_7q=[0.01  0.10], p8_9q=[0.01  0.08], p10q=3.00, p11_12_13q=[2.5  0.5  0.3], p15_17q=[4 1/89], p14_16q=[75.00  3], p18q=0, p19q=on}
      mask prompts: p3_4_5q "Power, Voltage and Frequency Ratings [MVA, kV, Hz]"; p6_7q "Stator Resistance Rs and Reactance Xs [p.u.  p.u.]"; p8_9q "Rotor Resitance Rr and Reactance Xr [p.u. p.u.]"; p10q "Magnetization Reactance Xm [p.u.]"; p11_12_13q "Inertia Constants Hwr Hm and Ks [kWs/kVA kWs/kVA p.u.]"; p15_17q "Number of poles p and gear box ratio [int  -]"; p14_16q "Blade length and number [m int]"; p18q "Number of machine that compose the park"; p19q "Connected"
      mask help: This block defines a constant speed wind turbine with third order asynchronous generator and dynamic shaft.
      mask init:
      | [x,y] = fm_draw('circle');
      | [xh,yh] = fm_draw('helix');
      mask Callback p19q: fm_block
      mask Display:
      | plot(1.4*x,1.4*y,[0,-2],[0 0],[-2 -3 -3 -2 -2],[-1 -1 1 1 -1],[-3 -5],[0 0],[1.4 3],[0 0],[2.2 2.2],[0 -1],[1.8 2.6],[-1 -1],[1.8 2.6],[-1.2 -1.2],[2.2 2.2],[-1.2 -2.2],[1.9 2.5],[-2.2 -2.2],[2.1 2.3],[-2.4 -2.4])
      | color('blue')
      | plot(x,y)
      | color('cyan')
      | plot(xh-4,3*yh)
  Ddsg : PMComponent  Tag=PSATblock  Description=Wind Turbines  PhysicalDomain=psatdomain  LeftPortType=p1  RightPortType=p1  LConnTagsString=__newl0  RConnTagsString=__newr0  mask(Ddsg){p3_4_5q=[2   25   60], p6q=0.01, p7_8q=[1  0.8], p9q=1.00, p10q=3, p11_12q=[10  3], p13_14q=[10  1], p15_16q=[0.01 0.01], p18_20q=[4 1/89], p17_19q=[75.00  3], p21_22q=[1.00  0.00], p23_24q=[0.7  -0.7], p25q=0, p26q=on}
      mask prompts: p3_4_5q "Power, Voltage and Frequency Ratings [MVA, kV, Hz]"; p6q "Stator Resistance Rs [p.u.]"; p7_8q "Direct and inverse reactances Xd and Xq [p.u.  p.u.]"; p9q "Constant field flux  Psi_p [p.u.]"; p10q "Inertia Constants Hm  [kWs/kVA]"; p11_12q "Pitch control gain and time constant  Kp, Tp [p.u.  s]"; p13_14q "Voltage control gain and time constant Kv  Tv [p.u.  s]"; p15_16q "Active and Reactive Power Control time constants Tep Teq [s s]"; p18_20q "Number of poles p and gear box ratio [int  -]"; p17_19q "Blade length and number [m int]"; p21_22q "Pmax and Pmin [p.u.  p.u.]"; p23_24q "Qmax and Qmin [p.u.  p.u.]"; p25q "Number of machines that compose the park"; p26q "Connected"
      mask help: This block defines a variable speed wind turbine with direct drive synchronous generator.
      mask init:
      | [x,y] = fm_draw('circle');
      | [xh,yh] = fm_draw('helix');
      mask Callback p26q: fm_block
      mask Display:
      | plot(1.4*x,1.4*y,[0,-2],[0 0],[-2 -3 -3 -2 -2],[-1 -1 1 1 -1],[-3 -5],[0 0],[1.4 2.075],[0 0],[3.95 4.5],[0 0])
      | plot(1.5*[0.3 0.3 -0.95 -0.95 0.3]+3.5,0.5*[-1.7 2.7  2.7  -1.7 -1.7]-0.25,1.5*[0 0.2]+3.5,0.5*[0.5 0.5]-0.25)
      | color('blue')
      | plot(x,y)
      | color('cyan')
      | plot(xh-4,3*yh)
      | color('magenta')
      | plot(1.5*[0 0]+3.5,0.5*[-0.5 1.5]-0.25,1.5*[0 -0.2]+3.5,0.5*[-0.5 -0.5]-0.25,1.5*[0 -0.65]+3.5,0.5*[1.5 1.5]-0.25)
      | plot(1.5*[-0.2 -0.2]+3.5,0.5*[-1 0]-0.25,1.5*[-0.2 -0.45]+3.5,0.5*[-1 -0.5]-0.25,1.5*[-0.2 -0.45]+3.5,0.5*[0 -0.5]-0.25,1.5*[-0.45 -0.45]+3.5,0.5*[-1 0]-0.25)
      | plot(1.5*[-0.2 -0.2]+3.5,0.5*[2 1]-0.25,1.5*[-0.45 -0.45]+3.5,0.5*[2 1]-0.25,1.5*[-0.45 -0.2]+3.5,0.5*[2 1.5]-0.25,1.5*[-0.45 -0.2]+3.5,0.5*[1 1.5]-0.25)
      | plot(1.5*[-0.65 -0.65]+3.5,0.5*[-0.5 1.5]-0.25,1.5*[-0.45 -0.65]+3.5,0.5*[-0.5 -0.5]-0.25,1.5*[-0.45 -0.65]+3.5,0.5*[1.5 1.5]-0.25)
      | plot(1.5*[-0.65 -0.85]+3.5,0.5*[0.5 0.5]-0.25,1.5*[-0.3 -0.3]+3.5,0.5*[1.7 2.2]-0.25,1.5*[-0.325 -0.275]+3.5,0.5*[1.975 1.975]-0.25)
  Dfig : PMComponent  Tag=PSATblock  Description=Wind Turbines  PhysicalDomain=psatdomain  LeftPortType=p1  RightPortType=p1  LConnTagsString=__newl0  RConnTagsString=__newr0  mask(Dfig){p3_4_5q=[2   25   60], p6_7q=[0.01  0.10], p8_9q=[0.01  0.08], p10q=3.00, p11q=3, p12_13q=[10 3], p14q=10, p15q=0.01, p17_19q=[4 1/89], p16_18q=[75.00  3], p20_21q=[1.00  0.00], p22_23q=[0.7  -0.7], p24q=1, p25q=on}
      mask prompts: p3_4_5q "Power, Voltage and Frequency Ratings [MVA, kV, Hz]"; p6_7q "Stator Resistance Rs and Reactance Xs [p.u.  p.u.]"; p8_9q "Rotor Resitance Rr and Reactance Xr [p.u. p.u.]"; p10q "Magnetization Reactance Xm [p.u.]"; p11q "Inertia Constants Hm  [kWs/kVA]"; p12_13q "Pitch control gain and time constant  Kp, Tp [p.u.  s]"; p14q "Voltage control gain Kv [p.u.]"; p15q "Power Control time constant Te [s]"; p17_19q "Number of poles p and gear box ratio [int  -]"; p16_18q "Blade length and number [m int]"; p20_21q "Pmax and Pmin [p.u.  p.u.]"; p22_23q "Qmax and Qmin [p.u.  p.u.]"; p24q "Number of wind generators that compose the park"; p25q "Connected"
      mask help: This block defines a variable speed wind turbine with doubly fed induction generator.
      mask init:
      | [x,y] = fm_draw('circle');
      | [xh,yh] = fm_draw('helix');
      mask Callback p25q: fm_block
      mask Display:
      | plot(1.4*x,1.4*y,[0,-2],[0 0],[-2 -3 -3 -2 -2],[-1 -1 1 1 -1],[-3 -5],[0 0],[1.4 3.5],[0 0],1,4.35,[0 0 1.075],[-1 -3.25 -3.25],[2.05  2.05],[0 -2.15])
      | plot(1.5*[0.3 0.3]+2.5,0.5*[-1.7 2.7]-3.5,1.5*[ -0.95  -0.95]+2.5,0.5*[-1.7 2.7]-3.5,1.5*[0 0.2]+2.5,0.5*[0.5 0.5]-3.5)
      | plot(1.5*[0.3 -0.95]+2.5,0.5*[2.7 2.7]-3.5,1.5*[0.3 -0.95]+2.5,0.5*[-1.7 -1.7]-3.5)
      | color('blue')
      | plot(x,y)
      | color('cyan')
      | plot(xh-4,3*yh)
      | color('magenta')
      | plot(1.5*[0 0]+2.5,0.5*[-0.5 1.5]-3.5,1.5*[0 -0.2]+2.5,0.5*[-0.5 -0.5]-3.5,1.5*[0 -0.65]+2.5,0.5*[1.5 1.5]-3.5)
      | plot(1.5*[-0.2 -0.2]+2.5,0.5*[-1 0]-3.5,1.5*[-0.2 -0.45]+2.5,0.5*[-1 -0.5]-3.5,1.5*[-0.2 -0.45]+2.5,0.5*[0 -0.5]-3.5,1.5*[-0.45 -0.45]+2.5,0.5*[-1 0]-3.5)
      | plot(1.5*[-0.2 -0.2]+2.5,0.5*[2 1]-3.5,1.5*[-0.45 -0.45]+2.5,0.5*[2 1]-3.5,1.5*[-0.45 -0.2]+2.5,0.5*[2 1.5]-3.5,1.5*[-0.45 -0.2]+2.5,0.5*[1 1.5]-3.5)
      | plot(1.5*[-0.65 -0.65]+2.5,0.5*[-0.5 1.5]-3.5,1.5*[-0.45 -0.65]+2.5,0.5*[-0.5 -0.5]-3.5,1.5*[-0.45 -0.65]+2.5,0.5*[1.5 1.5]-3.5)
      | plot(1.5*[-0.65 -0.85]+2.5,0.5*[0.5 0.5]-3.5,1.5*[-0.3 -0.3]+2.5,0.5*[1.7 2.2]-3.5,1.5*[-0.325 -0.275]+2.5,0.5*[1.975 1.975]-3.5)
  Wind : PMComponent  Tag=PSATblock  Description=Wind Turbines  PhysicalDomain=psatdomain  LeftPortType=p1  RightPortType=p1  RConnTagsString=__newr0  mask(Wind){out=1, p1q=measurements, p2q=15.00, p3q=1.225, p4q=4, p5q=0.1, p6_7q=[20  2], p8_9_10q=[5  15  1], p11_12_13q=[5  15  1], p14_15_16_17q=[50  0.01  0.2  50], p_18_19q=[10  1]}
      mask prompts: out "Number of output ports"; p1q "Wind model type"; p2q "Nominal wind speed [m/s]"; p3q "Air density rho [kg/m^3]"; p4q "Filter time constant tau [s]"; p5q "Sample time for wind measures [s]"; p6_7q "Weibull distribution constants  C and K"; p8_9_10q "Wind ramp constants Tsr, Ter and Awr [s s m/s]"; p11_12_13q "Wind gust constants Tsg, Teg and Awg [s s m/s]"; p14_15_16_17q "Wind turbolence constants h, z0, df and n [m - Hz int]"; p_18_19q "Mexican hat wavelet time center and shape factor"
      mask help: This block defines wind models for use with wind turbines.
      mask init:
      | fm_inout
      | [xa,ya] = fm_draw('arrow');
      mask TypeOptions p1q: measurements | weibull | composite | mexican_hat
      mask Display:
      | color('cyan')
      | plot(xa,ya,xa-0.2,ya-0.2,xa+0.2,ya+0.2,xa+0.4,ya+0.4,xa-0.4,ya-0.4)

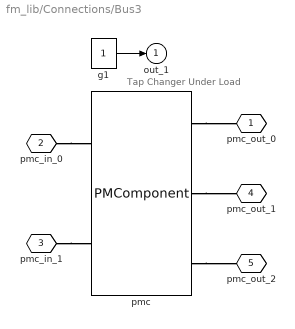
== system fm_lib/Connections/Bus3 ==
  note: Tap Changer Under Load
  g1 : Constant
  pmc : PMComponent  PhysicalDomain=psatdomain  LeftPortType=p1  RightPortType=p1  LConnTagsString=__newl0|__newl1  RConnTagsString=__newr0|__newr1|__newr2
  pmc_out_0 : PMIOPort  Tag=PMCPort  Port=1  Side=Left
  pmc_in_0 : PMIOPort  Tag=PMCPort  Port=2  Side=Right
  pmc_in_1 : PMIOPort  Port=3  Side=Right
  pmc_out_1 : PMIOPort  Port=4  Side=Left
  pmc_out_2 : PMIOPort  Port=5  Side=Left
  out_1 : Outport
  wires:
  g1/1 -> out_1/1
  connections:
  pmc_in_0/RConn1 -- pmc/LConn1
  pmc/RConn1 -- pmc_out_0/RConn1
  pmc_in_1/RConn1 -- pmc/LConn2
  pmc/RConn2 -- pmc_out_1/RConn1
  pmc/RConn3 -- pmc_out_2/RConn1

== system fm_lib/Connections/Link1 ==
  note: Link
  Enable : EnablePort
  Atomic Subsystem : PMComponent  PhysicalDomain=psatdomain  LeftPortType=p1  RightPortType=p1  LConnTagsString=__newl0  RConnTagsString=__newr0
  Connection Port : PMIOPort  Tag=PMCPort  Port=1  Side=Left
  Connection Port1 : PMIOPort  Tag=PMCPort  Port=2  Side=Right
  connections:
  Connection Port/RConn1 -- Atomic Subsystem/LConn1
  Atomic Subsystem/RConn1 -- Connection Port1/RConn1

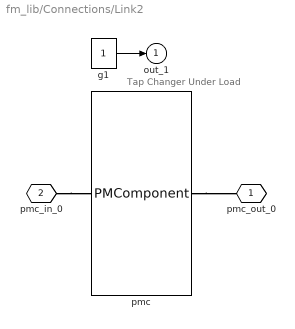
== system fm_lib/Connections/Link2 ==
  note: Tap Changer Under Load
  g1 : Constant
  pmc : PMComponent  PhysicalDomain=psatdomain  LeftPortType=p1  RightPortType=p1  LConnTagsString=__newl0  RConnTagsString=__newr0
  pmc_out_0 : PMIOPort  Tag=PMCPort  Port=1  Side=Left
  pmc_in_0 : PMIOPort  Tag=PMCPort  Port=2  Side=Right
  out_1 : Outport
  wires:
  g1/1 -> out_1/1
  connections:
  pmc/RConn1 -- pmc_out_0/RConn1
  pmc_in_0/RConn1 -- pmc/LConn1

== system fm_lib/Connections/Varname ==

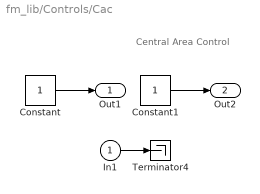
== system fm_lib/Controls/Cac ==
  note: Central Area Control
  In1 : Inport
  Constant : Constant
  Constant1 : Constant
  Terminator4 : Terminator
  Out1 : Outport
  Out2 : Outport  Port=2
  wires:
  Constant1/1 -> Out2/1
  In1/1 -> Terminator4/1
  Constant/1 -> Out1/1

== system fm_lib/Controls/Cluster ==
  note: Cluster Controller
  In1 : Inport
  Constant : Constant
  Terminator4 : Terminator
  Out1 : Outport
  wires:
  In1/1 -> Terminator4/1
  Constant/1 -> Out1/1

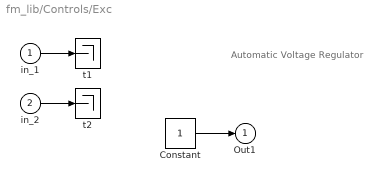
== system fm_lib/Controls/Exc ==
  note: Automatic Voltage Regulator
  in_1 : Inport
  in_2 : Inport  Port=2
  Constant : Constant
  t1 : Terminator
  t2 : Terminator
  Out1 : Outport
  wires:
  Constant/1 -> Out1/1
  in_1/1 -> t1/1
  in_2/1 -> t2/1

== system fm_lib/Controls/Oxl ==
  note: Overexcitation
      | Limiter
  Constant : Constant
  Out1 : Outport
  wires:
  Constant/1 -> Out1/1

== system fm_lib/Controls/Pod ==
  note: Suplementary Stabilizing Control Loop for SVCs
  In1 : Inport
  Constant : Constant
  Terminator4 : Terminator
  Out1 : Outport
  wires:
  In1/1 -> Terminator4/1
  Constant/1 -> Out1/1

== system fm_lib/Controls/Pss ==
  note: Power System Stabilizer
  Constant : Constant
  Out1 : Outport
  wires:
  Constant/1 -> Out1/1

== system fm_lib/Controls/Tg ==
  note: Turbine Governor
  Constant : Constant
  Out1 : Outport
  wires:
  Constant/1 -> Out1/1

== system fm_lib/Machines/Syn ==
  note: Synchronous Machine
  Atomic Subsystem : PMComponent  PhysicalDomain=psatdomain  LeftPortType=p1  RightPortType=p1  RConnTagsString=__newr0
  Connection Port1 : PMIOPort  Tag=PMCPort  Port=1  Side=Right
  connections:
  Atomic Subsystem/RConn1 -- Connection Port1/RConn1

== system fm_lib/OPF & CPF/Ypdp ==

== system fm_lib/OPF & CPF/Ypdp1 ==

== system fm_lib/Others/Mass ==
  note: Dynamic Shaft
  Constant : Constant
  Out1 : Outport
  wires:
  Constant/1 -> Out1/1

== system fm_lib/ULTC/Ltc ==
  note: Tap Changer Under Load
  Atomic Subsystem : PMComponent  PhysicalDomain=psatdomain  LeftPortType=p1  RightPortType=p1  LConnTagsString=__newl0  RConnTagsString=__newr0
  Connection Port1 : PMIOPort  Tag=PMCPort  Port=1  Side=Left
  Connection Port2 : PMIOPort  Tag=PMCPort  Port=2  Side=Right
  connections:
  Atomic Subsystem/RConn1 -- Connection Port1/RConn1
  Connection Port2/RConn1 -- Atomic Subsystem/LConn1

== system fm_lib/ULTC/Ltc1 ==
  note: Tap Changer Under Load
  in_2 : EnablePort
  Atomic Subsystem : PMComponent  PhysicalDomain=psatdomain  LeftPortType=p1  RightPortType=p1  LConnTagsString=__newl0  RConnTagsString=__newr0
  Connection Port1 : PMIOPort  Tag=PMCPort  Port=1  Side=Left
  Connection Port2 : PMIOPort  Tag=PMCPort  Port=2  Side=Right
  connections:
  Connection Port2/RConn1 -- Atomic Subsystem/LConn1
  Atomic Subsystem/RConn1 -- Connection Port1/RConn1
